simulink model "psk_pe_est"  (Simulink 8.7)
settings: Solver=FixedStepDiscrete  SolverMode=SingleTasking  StartTime=0.0  StopTime=5  FixedStep=1/100000  RelTol=1e-3  AbsTol=1e-6
libraries: commchan3 x1, commsink2 x1, commfilt2 x1, dspsrcs4 x1
settings Model: Creator=amoura  LastModifiedBy=Artur Moura
settings DataIOCC: LimitDataPoints=off  SignalLoggingSaveFormat=ModelDataLogs
settings OptimizationCC: BlockReduction=off  BooleanDataType=off  ExpressionDepthLimit=2147483647  InitFltsAndDblsToZero=on
settings DebuggingCC: SaveWithParameterizedLinksMsg=none  SignalResolutionControl=TryResolveAllWithWarning  MultiTaskDSMMsg=warning  MultiTaskCondExecSysMsg=none  FcnCallInpInsideContextMsg=UseLocalSettings  StateNameClashWarn=warning
settings HardwareCC: TargetUnknown=on
settings RTWCC: TemplateMakefile=grt_unix.tmf
settings GRTTargetCC: TargetFcnLib=ansi_tfl_tmw.mat  ModelReferenceCompliant=off  CombineOutputUpdateFcns=off  MatFileLogging=off  GRTInterface=on

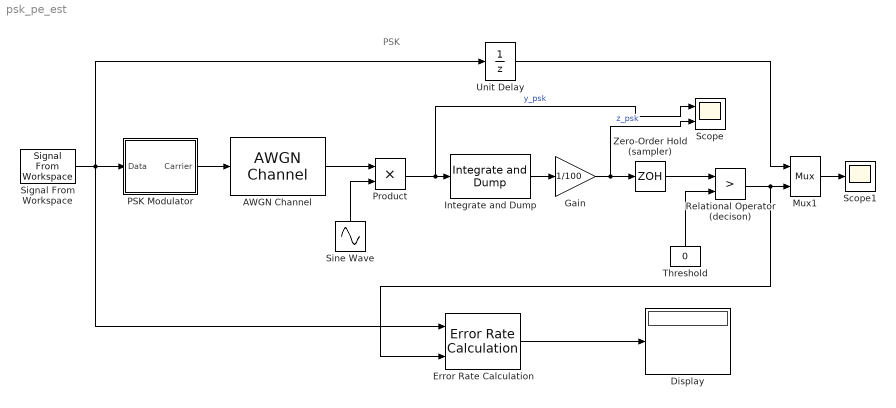
== system psk_pe_est ==
  note: PSK
  AWGN Channel : commchan3/AWGN Channel  InputProcessing=Inherited (this choice will be removed - see release notes)  seed=67  noiseMode=Variance from mask  EbNodB=0  EsNodB=10  SNRdB=10  bitsPerSym=1  Ps=.5/1000  Tsym=1/1000  variance=10
  Display : Display
  Error Rate Calculation : commsink2/Error Rate Calculation  N=1  st_delay=0  cp_mode=Entire frame  subframe=[]  PMode=Port  WsName=ErrorVec  RsMode2=off  stop=off  numErr=100  maxBits=1e6
  Gain : Gain  Gain=1/100  SampleTime=1/100000  SaturateOnIntegerOverflow=on  OutDataTypeStr=Inherit: Same as input  ParamDataTypeStr=Inherit: Same as input
  Integrate and Dump : commfilt2/Integrate and Dump  obssamples=100  offsetsamples=1  nodump=on  roundingMode=Floor  overflowMode=off  outputDataTypeStr=Inherit: Same as accumulator  outputLastDataTypeStr=Inherit: Same as accumulator
  Mux1 : Mux  Inputs=2
  PSK Modulator : Subsystem
  Product : Product  SampleTime=1/100000  SaturateOnIntegerOverflow=on  RndMeth=Zero  InputSameDT=on  OutDataTypeStr=Inherit: Same as first input
  Relational Operator (decison) : RelationalOperator  Operator=>  InputSameDT=on
  Scope : Scope  NumInputPorts=2
  Scope1 : Scope
  Signal From Workspace : dspsrcs4/Signal From Workspace  X=randi([0 1],10000,1)  Ts=1/1000  nsamps=1  OutputAfterFinalValue=Cyclic repetition  ignoreOrWarnInputAndFrameLengths=off  OutputFrames=on
  Sine Wave : Sin  Frequency=2*pi*10000  SampleTime=0
  Threshold : Constant  Value=0
  Unit Delay : UnitDelay  SampleTime=1/1000
  Zero-Order Hold (sampler) : ZeroOrderHold  SampleTime=1/1000
  wires:
  PSK Modulator/1(Carrier) -> AWGN Channel/1
  Unit Delay/1 -> Mux1/1
  Relational Operator (decison)/1 -> Mux1/2, Error Rate Calculation/2
  Mux1/1 -> Scope1/1
  Gain/1 -> Zero-Order Hold (sampler)/1, Scope/2  "z_psk"
  Zero-Order Hold (sampler)/1 -> Relational Operator (decison)/1
  Product/1 -> Integrate and Dump/1, Scope/1  "y_psk"
  AWGN Channel/1 -> Product/1
  Signal From Workspace/1 -> Unit Delay/1, PSK Modulator/1(Data), Error Rate Calculation/1
  Integrate and Dump/1 -> Gain/1
  Threshold/1 -> Relational Operator (decison)/2
  Sine Wave/1 -> Product/2
  Error Rate Calculation/1 -> Display/1

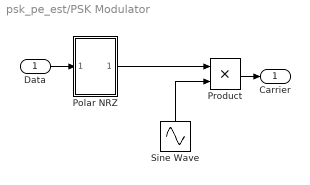
== system psk_pe_est/PSK Modulator ==
  Data : Inport
  Polar NRZ : Subsystem  mask(Polar NRZ){}
      mask help:
      | This block encodes a unipolar NRZ signal into the polar NRZ line code
      |
      | The output values are +1 for a nonzero input and -1 for a zero one.
      mask Display: disp('Polar\nNRZ')
  Product : Product  SaturateOnIntegerOverflow=on  RndMeth=Zero  InputSameDT=on  OutDataTypeStr=Inherit: Same as first input
  Sine Wave : Sin  Frequency=2*pi*10000  SampleTime=0
  Carrier : Outport  InitialOutput=0
  wires:
  Polar NRZ/1(Out1) -> Product/1
  Sine Wave/1 -> Product/2
  Data/1 -> Polar NRZ/1(In1)
  Product/1 -> Carrier/1

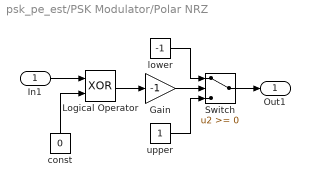
== system psk_pe_est/PSK Modulator/Polar NRZ ==
  In1 : Inport
  Gain : Gain  Gain=-1  SaturateOnIntegerOverflow=on  OutDataTypeStr=Inherit: Same as input  ParamDataTypeStr=Inherit: Same as input
  Logical Operator : Logic  Operator=XOR
  Switch : Switch  SaturateOnIntegerOverflow=on  InputSameDT=on
  const : Constant  Value=0
  lower : Constant  Value=-1
  upper : Constant
  Out1 : Outport  InitialOutput=0
  wires:
  const/1 -> Logical Operator/2
  Logical Operator/1 -> Gain/1
  Switch/1 -> Out1/1
  Gain/1 -> Switch/2
  upper/1 -> Switch/3
  lower/1 -> Switch/1
  In1/1 -> Logical Operator/1
